simulink model "MPC_point_5_oldversion"  (R2021b)
settings: Solver=VariableStepAuto  StartTime=0.0  StopTime=T_sim  RelTol=1e-3
values from neighbouring files (symbols this model uses):
  C = [0       1      0  0 ... (first row only)    [main.m]
  C_states = eye(length(A))    [main.m]
  D_states = zeros(length(B), 1)    [main.m]
  N5 = 100    [main.m]
  Q5 = Q_d    [main.m]
  R5 = R_d    (= 10000)    [main.m]
  S5 = P_d    [main.m]
  sysd = c2d(sys,T_sampling)    [main.m]
  T_sampling = 2*pi/omega_sampling    [main.m]
  u_max = deg2rad(15)    [main.m]
  u_min = deg2rad(-15)    [main.m]
  x0 = [deg2rad(0) deg2rad(15) 0 -300]    [main.m]
  x2_max = deg2rad(20)    [main.m]
  x2_min = deg2rad(-20)    [main.m]
  x_ref = [0 0 0 0]    [main.m]
undefined symbols (not defined in the file or in its folder): Klqr_d, mpc_point_3, mpc_point_5, mpc_point_6, mpc_point_7, over_shot, slewratemax, slewratemin, start_sign
settings Model: Creator=PaoloA  LastModifiedBy=PaoloA

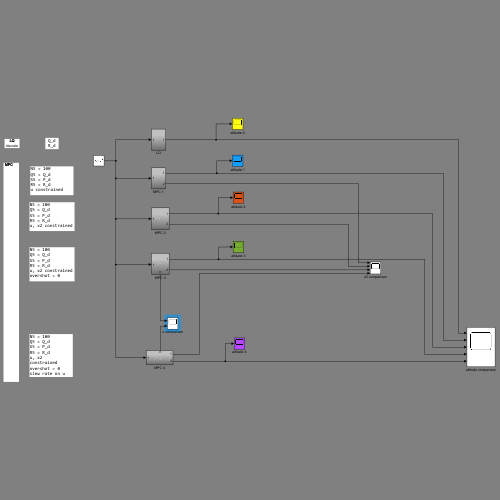
[thumbnail: Simulink's stored preview of the top-level diagram]
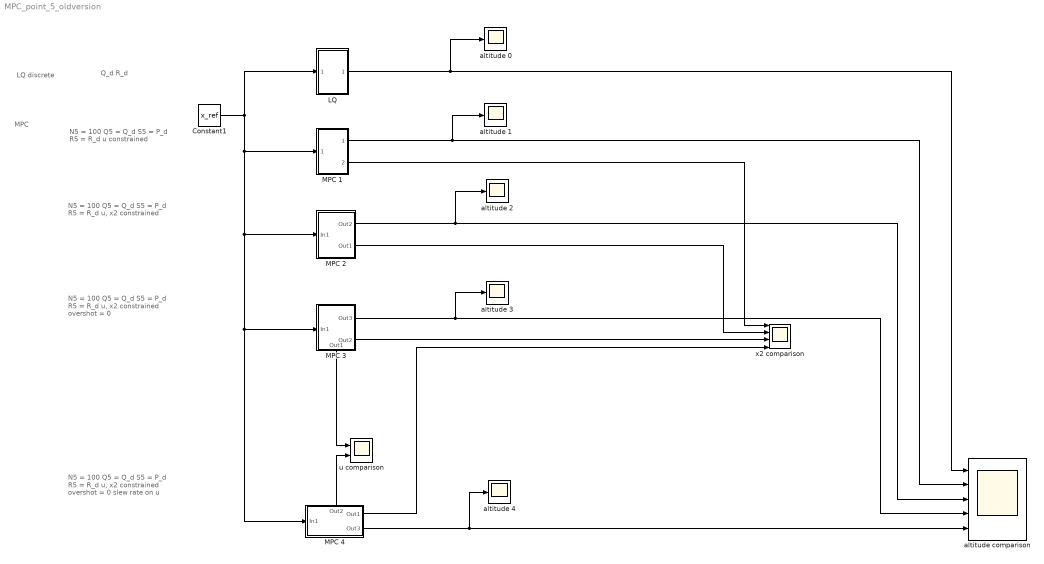
== system MPC_point_5_oldversion ==
  note: MPC
  note: N5 = 100
      | Q5 = Q_d
      | S5 = P_d
      | R5 = R_d
      | u, x2 constrained
  note: N5 = 100
      | Q5 = Q_d
      | S5 = P_d
      | R5 = R_d
      | u constrained
  note: LQ
      | discrete
  note: Q_d
      | R_d
  note: N5 = 100
      | Q5 = Q_d
      | S5 = P_d
      | R5 = R_d
      | u, x2 constrained
      | overshot = 0
  note: N5 = 100
      | Q5 = Q_d
      | S5 = P_d
      | R5 = R_d
      | u, x2 constrained
      | overshot = 0
      | slew rate on u
  Constant1 : Constant  Value=x_ref
  LQ : Subsystem
  MPC 1 : Subsystem
  MPC 2 : Subsystem
  MPC 3 : Subsystem
      settings: PortSchema="{\"entries\":[{\"content\":{\"sides\":[{\"content\":{\"connectorIds\":[\"In1\"]},\"type\":\"ConnectorPlacement.EquallySpacedRectSide\",\"uuid\":\"3ba6209e-b61b-449f-a4a5-696b47182f55\"},{\"content\":{\"connectorIds\":[\"Out1\",\"Out2\"],\"side\":\"RIGHT\"},\"type\":\"ConnectorPlacement.EquallySpacedRectSide\",\"uuid\":\"4a483f9f-8e08-4e29-ae4e-907177901594\"},{\"content\":{\"connectorIds\":[],\"side\":\"TOP\"},\"type\":\"ConnectorPlacement.EquallySpacedRectSide\",\"uuid\":\"39de9f9a-29a6-4241-8c9a-519bdf7c185a\"},{\"content\":{\"connectorIds\":[\"Out3\"],\"side\":\"BOTTOM\"},\"type\":\"ConnectorPlacement.EquallySpacedRectSide\",\"uuid\":\"7bc8ee22-34f5-4f07-9884-f0865d7ca937\"}]},\"type\":\"ConnectorPlacement.EquallySpacedConnector\",\"uuid\":\"5a1fb1b5-a7a5-4102-96c4-e89226b1c69b\"}],\"packageUris\":[\"http://schema.mathworks.com/mf0/Connector/R2020b\"],\"version\":\"1.0\"}"
  MPC 4 : Subsystem
      settings: PortSchema="{\"entries\":[{\"content\":{\"sides\":[{\"content\":{\"connectorIds\":[\"In1\"]},\"type\":\"ConnectorPlacement.EquallySpacedRectSide\",\"uuid\":\"3ba6209e-b61b-449f-a4a5-696b47182f55\"},{\"content\":{\"connectorIds\":[\"Out1\",\"Out2\"],\"side\":\"RIGHT\"},\"type\":\"ConnectorPlacement.EquallySpacedRectSide\",\"uuid\":\"4a483f9f-8e08-4e29-ae4e-907177901594\"},{\"content\":{\"connectorIds\":[\"Out3\"],\"side\":\"TOP\"},\"type\":\"ConnectorPlacement.EquallySpacedRectSide\",\"uuid\":\"39de9f9a-29a6-4241-8c9a-519bdf7c185a\"}]},\"type\":\"ConnectorPlacement.EquallySpacedConnector\",\"uuid\":\"5a1fb1b5-a7a5-4102-96c4-e89226b1c69b\"}],\"packageUris\":[\"http://schema.mathworks.com/mf0/Connector/R2020b\"],\"version\":\"1.0\"}"
  altitude {0..4} (5 alike) : Scope
  altitude comparison : Scope  NumInputPorts=5
  u comparison : Scope  NumInputPorts=2
  x2 comparison : Scope  NumInputPorts=4
  wires:
  LQ/1(Out1) -> altitude comparison/1, altitude 0/1
  MPC 1/1(Out2) -> altitude 1/1, altitude comparison/2
  MPC 1/2(Out1) -> x2 comparison/1
  MPC 2/1(Out2) -> altitude comparison/3, altitude 2/1
  MPC 2/2(Out1) -> x2 comparison/2
  MPC 4/2(Out3) -> altitude comparison/5, altitude 4/1
  MPC 4/1(Out1) -> x2 comparison/4
  MPC 4/3(Out2) -> u comparison/2
  Constant1/1 -> MPC 4/1(In1), MPC 3/1(In1), MPC 2/1(In1), MPC 1/1(In1), LQ/1(In1)
  MPC 3/1(Out3) -> altitude comparison/4, altitude 3/1
  MPC 3/2(Out2) -> x2 comparison/3
  MPC 3/3(Out1) -> u comparison/1

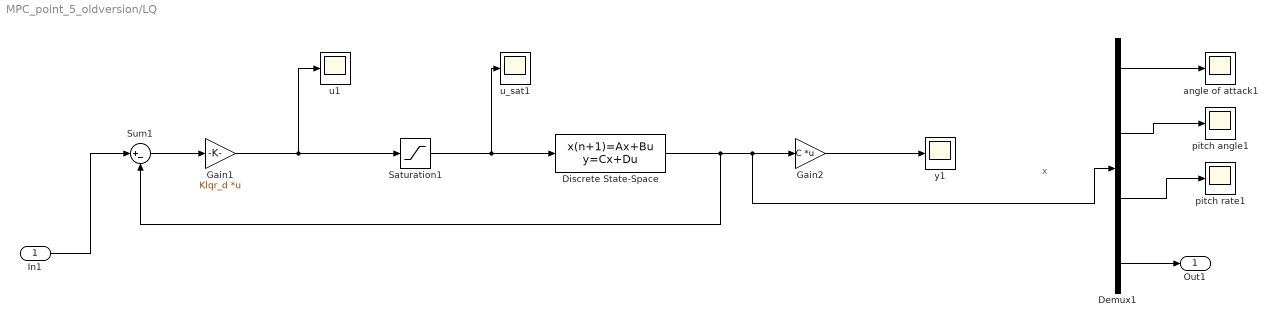
== system MPC_point_5_oldversion/LQ ==
  note: x
  In1 : Inport
  Demux1 : Demux
  Discrete State-Space : DiscreteStateSpace  A=sysd.A  B=sysd.B  C=C_states  D=D_states  InitialCondition=x0  SampleTime=T_sampling
  Gain1 : Gain  Gain=Klqr_d  Multiplication=Matrix(K*u)
  Gain2 : Gain  Gain=C  Multiplication=Matrix(K*u)
  Saturation1 : Saturate  UpperLimit=u_max  LowerLimit=u_min
  Sum1 : Sum  Inputs=|+-
  angle of attack1 : Scope
  pitch angle1 : Scope
  pitch rate1 : Scope
  u1 : Scope
  u_sat1 : Scope
  y1 : Scope
  Out1 : Outport
  wires:
  Gain2/1 -> y1/1
  Discrete State-Space/1 -> Demux1/1, Gain2/1, Sum1/2
  Saturation1/1 -> Discrete State-Space/1, u_sat1/1
  Gain1/1 -> u1/1, Saturation1/1
  Demux1/4 -> Out1/1
  Demux1/1 -> angle of attack1/1
  Sum1/1 -> Gain1/1
  Demux1/2 -> pitch angle1/1
  Demux1/3 -> pitch rate1/1
  In1/1 -> Sum1/1

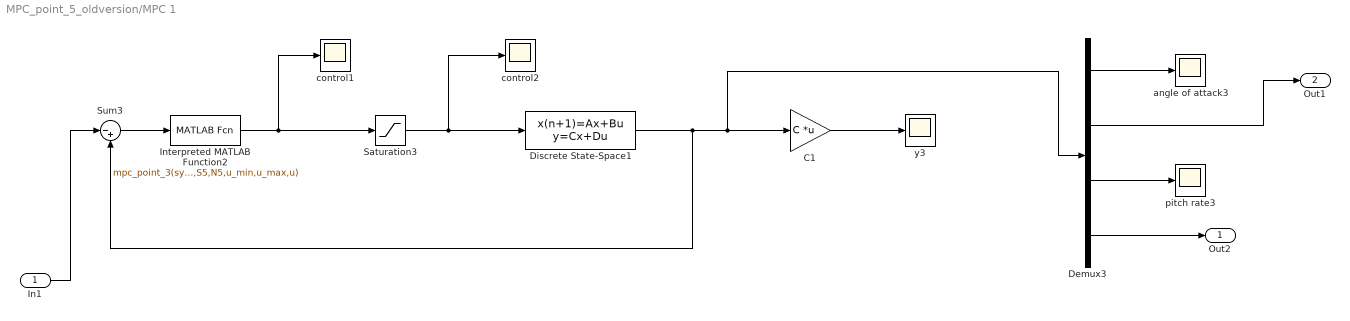
== system MPC_point_5_oldversion/MPC 1 ==
  In1 : Inport
  C1 : Gain  Gain=C  Multiplication=Matrix(K*u)
  Demux3 : Demux
  Discrete State-Space1 : DiscreteStateSpace  A=sysd.A  B=sysd.B  C=C_states  D=D_states  InitialCondition=x0  SampleTime=T_sampling
  Interpreted MATLAB Function2 : MATLABFcn  MATLABFcn=mpc_point_3(sysd.A,sysd.B,Q5,R5,S5,N5,u_min,u_max,u)  OutputDimensions=1
  Saturation3 : Saturate  UpperLimit=u_max  LowerLimit=u_min
  Sum3 : Sum  Inputs=|-+
  angle of attack3 : Scope
  control1 : Scope
  control2 : Scope
  pitch rate3 : Scope
  y3 : Scope
  Out2 : Outport
  Out1 : Outport  Port=2
  wires:
  C1/1 -> y3/1
  Interpreted MATLAB Function2/1 -> Saturation3/1, control1/1
  Demux3/1 -> angle of attack3/1
  Discrete State-Space1/1 -> C1/1, Demux3/1, Sum3/2
  Demux3/4 -> Out2/1
  Saturation3/1 -> Discrete State-Space1/1, control2/1
  Sum3/1 -> Interpreted MATLAB Function2/1
  Demux3/3 -> pitch rate3/1
  In1/1 -> Sum3/1
  Demux3/2 -> Out1/1

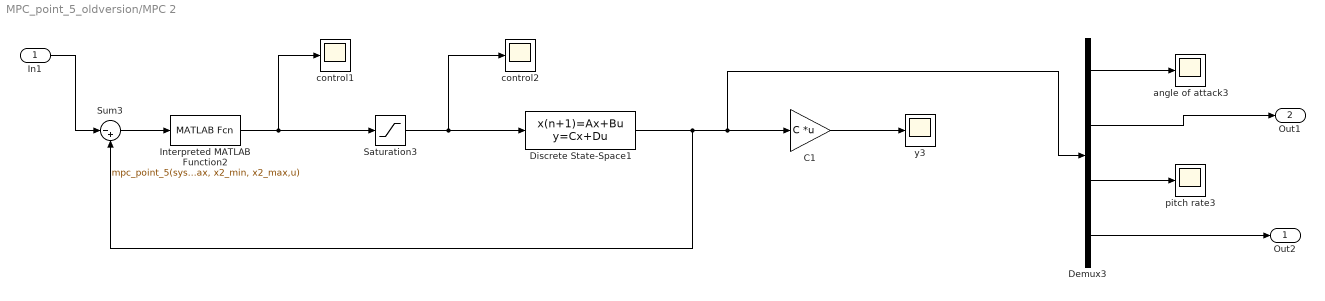
== system MPC_point_5_oldversion/MPC 2 ==
  In1 : Inport
  C1 : Gain  Gain=C  Multiplication=Matrix(K*u)
  Demux3 : Demux
  Discrete State-Space1 : DiscreteStateSpace  A=sysd.A  B=sysd.B  C=C_states  D=D_states  InitialCondition=x0  SampleTime=T_sampling
  Interpreted MATLAB Function2 : MATLABFcn  MATLABFcn=mpc_point_5(sysd.A,sysd.B,Q5,R5,S5,N5,u_min,u_max, x2_min, x2_max,u)  OutputDimensions=1
  Saturation3 : Saturate  UpperLimit=u_max  LowerLimit=u_min
  Sum3 : Sum  Inputs=|-+
  angle of attack3 : Scope
  control1 : Scope
  control2 : Scope
  pitch rate3 : Scope
  y3 : Scope
  Out2 : Outport
  Out1 : Outport  Port=2
  wires:
  Interpreted MATLAB Function2/1 -> Saturation3/1, control1/1
  Demux3/1 -> angle of attack3/1
  Saturation3/1 -> Discrete State-Space1/1, control2/1
  Sum3/1 -> Interpreted MATLAB Function2/1
  C1/1 -> y3/1
  Demux3/3 -> pitch rate3/1
  Discrete State-Space1/1 -> C1/1, Demux3/1, Sum3/2
  In1/1 -> Sum3/1
  Demux3/2 -> Out1/1
  Demux3/4 -> Out2/1

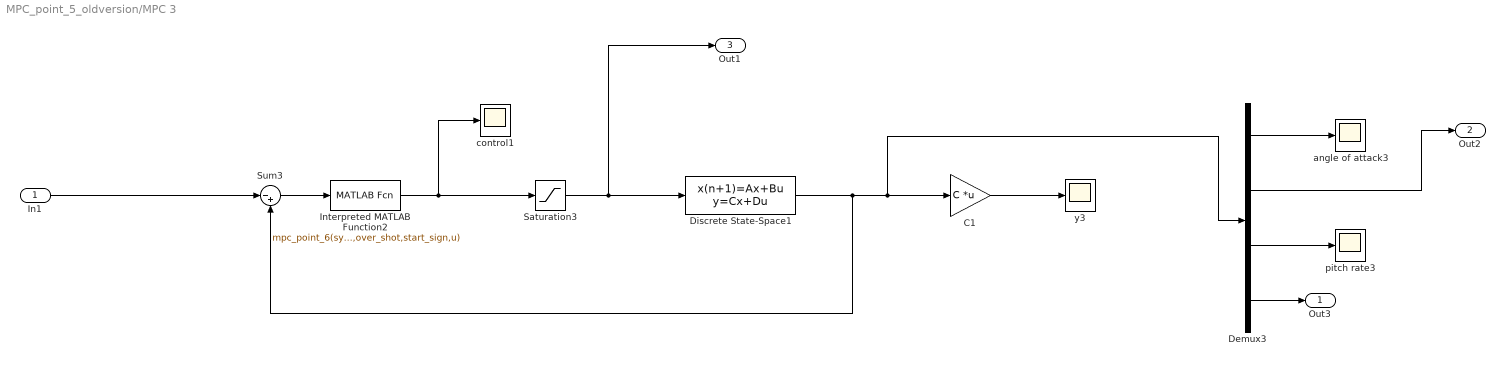
== system MPC_point_5_oldversion/MPC 3 ==
  In1 : Inport
  C1 : Gain  Gain=C  Multiplication=Matrix(K*u)
  Demux3 : Demux
  Discrete State-Space1 : DiscreteStateSpace  A=sysd.A  B=sysd.B  C=C_states  D=D_states  InitialCondition=x0  SampleTime=T_sampling
  Interpreted MATLAB Function2 : MATLABFcn  MATLABFcn=mpc_point_6(sysd.A,sysd.B,Q5,R5,S5,N5,u_min,u_max, x2_min, x2_max,over_shot,start_sign,u)  OutputDimensions=1
  Saturation3 : Saturate  UpperLimit=u_max  LowerLimit=u_min
  Sum3 : Sum  Inputs=|-+
  angle of attack3 : Scope
  control1 : Scope
  pitch rate3 : Scope
  y3 : Scope
  Out3 : Outport
  Out2 : Outport  Port=2
  Out1 : Outport  Port=3
  wires:
  Demux3/4 -> Out3/1
  Demux3/1 -> angle of attack3/1
  Discrete State-Space1/1 -> C1/1, Demux3/1, Sum3/2
  In1/1 -> Sum3/1
  Sum3/1 -> Interpreted MATLAB Function2/1
  C1/1 -> y3/1
  Demux3/3 -> pitch rate3/1
  Saturation3/1 -> Out1/1, Discrete State-Space1/1
  Interpreted MATLAB Function2/1 -> Saturation3/1, control1/1
  Demux3/2 -> Out2/1

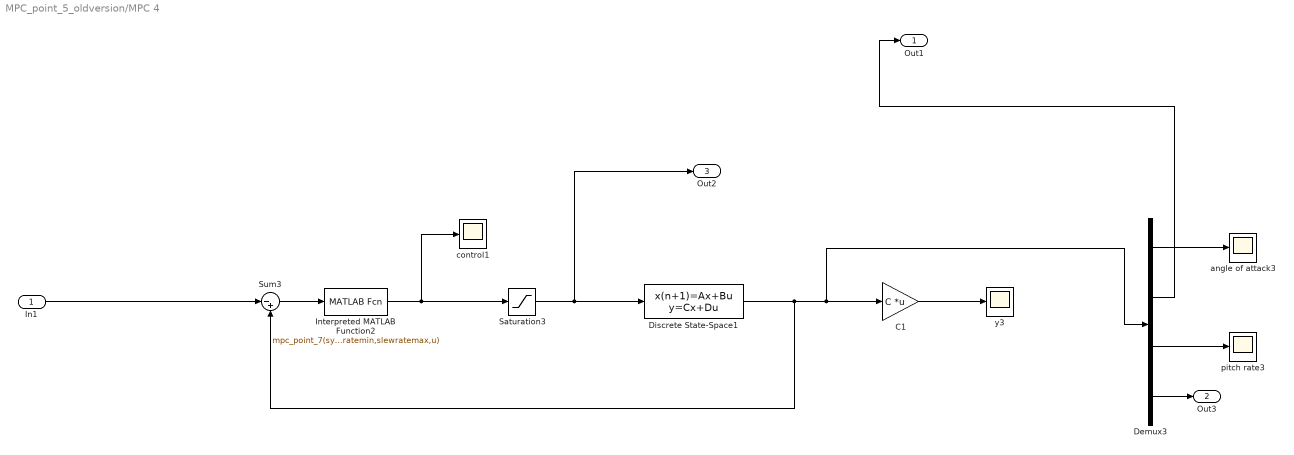
== system MPC_point_5_oldversion/MPC 4 ==
  In1 : Inport
  C1 : Gain  Gain=C  Multiplication=Matrix(K*u)
  Demux3 : Demux
  Discrete State-Space1 : DiscreteStateSpace  A=sysd.A  B=sysd.B  C=C_states  D=D_states  InitialCondition=x0  SampleTime=T_sampling
  Interpreted MATLAB Function2 : MATLABFcn  MATLABFcn=mpc_point_7(sysd.A,sysd.B,Q5,R5,S5,N5,u_min,u_max, x2_min, x2_max,over_shot,start_sign,slewratemin,slewratemax,u)  OutputDimensions=1
  Saturation3 : Saturate  UpperLimit=u_max  LowerLimit=u_min
  Sum3 : Sum  Inputs=|-+
  angle of attack3 : Scope
  control1 : Scope
  pitch rate3 : Scope
  y3 : Scope
  Out1 : Outport
  Out3 : Outport  Port=2
  Out2 : Outport  Port=3
  wires:
  Discrete State-Space1/1 -> C1/1, Demux3/1, Sum3/2
  Demux3/1 -> angle of attack3/1
  Demux3/3 -> pitch rate3/1
  Interpreted MATLAB Function2/1 -> Saturation3/1, control1/1
  Saturation3/1 -> Out2/1, Discrete State-Space1/1
  Sum3/1 -> Interpreted MATLAB Function2/1
  C1/1 -> y3/1
  Demux3/2 -> Out1/1
  Demux3/4 -> Out3/1
  In1/1 -> Sum3/1
